simulink model "Suspension_model"  (R2020b)
settings: Solver=VariableStepAuto  StartTime=0.0  StopTime=10.0  RelTol=1e-3
undefined symbols (not defined in the file): b1, b2, k1, k2, m1, m2
settings Model: Creator=Avengers  LastModifiedBy=Avengers

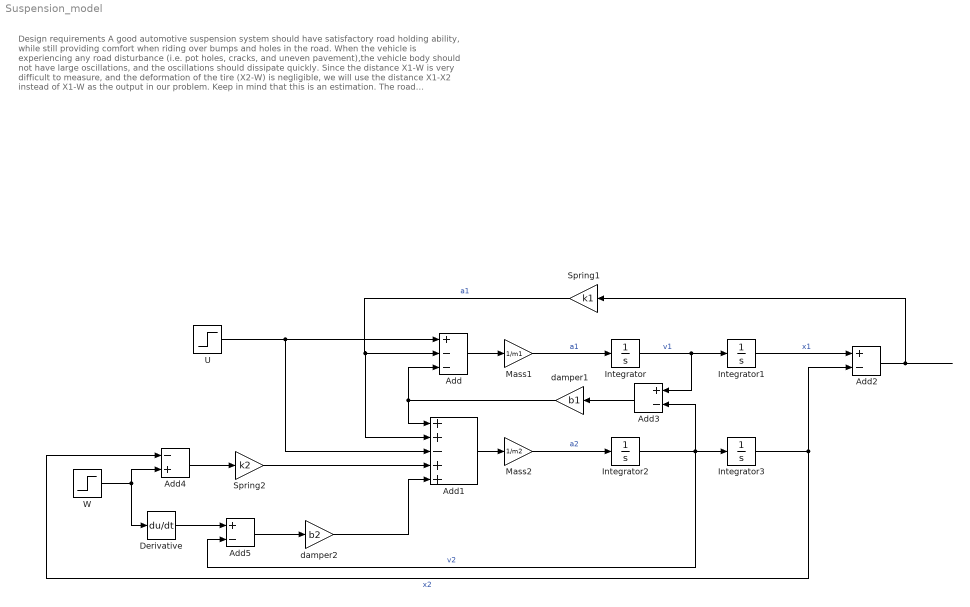
== system Suspension_model ==
  note: Design requirements
      | A good automotive suspension system should have satisfactory road holding ability, while still providing comfort when riding over bumps and holes in the road. When the vehicle is experiencing any road disturbance (i.e. pot holes, cracks, and uneven pavement),the vehicle body should not have large oscillations, and the oscillations should dissipate quickly. Since the distance X1-W is very difficult to measure, and the deformation of the tire (X2-W) is negligible, we will use the distance X1-X2 instead of X1-W as the output in our problem. Keep in mind that this is an estimation.
      | The road disturbance (W) in this problem will be simulated by a step input. This step could represent the vehicle coming out of a pothole. We want to design a feedback controller so that the output (X1-X2) has an overshoot less than 5% and a settling time shorter than 5 seconds. For example, when the vehicle runs onto a 10 cm high step, the vehicle body will oscillate within a range of +/- 5 mm and return to a smooth ride within 5 seconds.
  Add : Sum  Inputs=+--
  Add1 : Sum  Inputs=++-++
  Add2 : Sum  Inputs=+-
  Add3 : Sum  Inputs=+-
  Add4 : Sum  Inputs=-+
  Add5 : Sum  Inputs=+-
  Derivative : Derivative
  Integrator{,1..3} (4 alike) : Integrator
  Mass1 : Gain  Gain=1/m1
  Mass2 : Gain  Gain=1/m2
  Spring1 : Gain  Gain=k1
  Spring2 : Gain  Gain=k2
  U : Step  Time=0  SampleTime=0
  W : Step  Time=0  After=0  SampleTime=0
  damper1 : Gain  Gain=b1
  damper2 : Gain  Gain=b2
  wires:
  Integrator/1 -> Add3/1, Integrator1/1  "v1"
  Mass1/1 -> Integrator/1  "a1"
  Integrator1/1 -> Add2/1  "x1"
  Integrator3/1 -> Add2/2, Add4/1  "x2"
  Mass2/1 -> Integrator2/1  "a2"
  Add/1 -> Mass1/1
  Add1/1 -> Mass2/1
  Add2/1 -> Spring1/1
  Spring1/1 -> Add1/2, Add/2  "a1"
  Add3/1 -> damper1/1
  damper1/1 -> Add1/1, Add/3
  Add4/1 -> Spring2/1
  Spring2/1 -> Add1/4
  damper2/1 -> Add1/5
  Add5/1 -> damper2/1
  W/1 -> Add4/2, Derivative/1
  Integrator2/1 -> Add5/2, Add3/2, Integrator3/1  "v2"
  Derivative/1 -> Add5/1
  U/1 -> Add1/3, Add/1
